simulink model "ModeleVehicule"  (R2018a)
settings: Solver=VariableStepAuto  StartTime=0.0  StopTime=1180  RelTol=1e-3
undefined symbols (not defined in the file or in its folder): cb, crr, cx, g, m, mlimit, nc, nm, nr, r, rho, rr, s
libraries: drivecyclelib x1
settings Model: Creator=Thomas  LastModifiedBy=Thomas

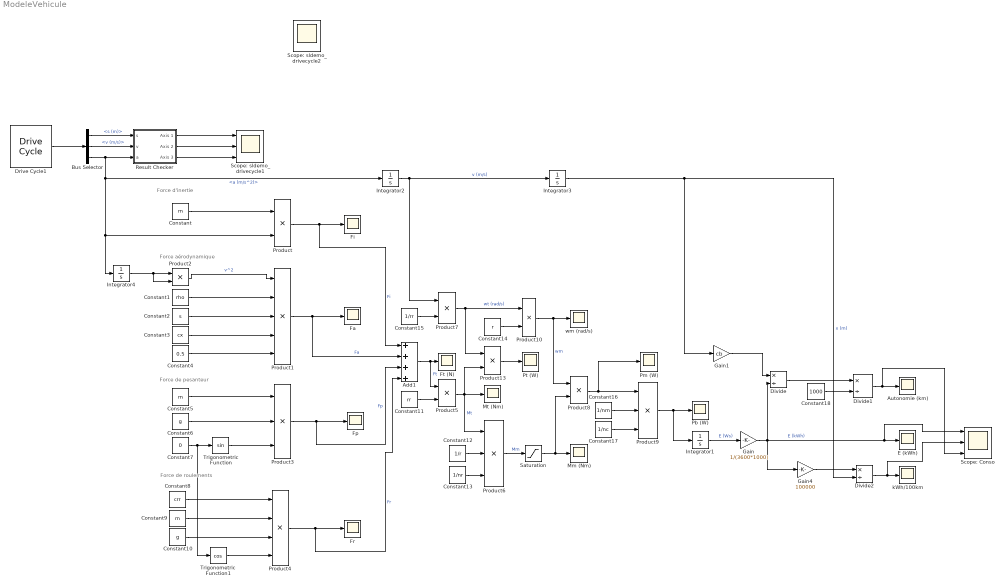
== system ModeleVehicule ==
  note: Force de pesanteur
  note: Force aérodynamique
  note: Force d'inertie
  note: Force de roulements
  Add1 : Sum  Inputs=++++
  Autonomie (km) : Scope
  Bus Selector : BusSelector  OutputSignals=s (m),v (m/s),a (m/s^2)
  Constant : Constant  Value=m
  Constant1 : Constant  Value=rho
  Constant10 : Constant  Value=g
  Constant11 : Constant  Value=rr
  Constant12 : Constant  Value=1/r
  Constant13 : Constant  Value=1/nr
  Constant14 : Constant  Value=r
  Constant15 : Constant  Value=1/rr
  Constant16 : Constant  Value=1/nm
  Constant17 : Constant  Value=1/nc
  Constant18 : Constant  Value=1000
  Constant2 : Constant  Value=s
  Constant3 : Constant  Value=cx
  Constant4 : Constant  Value=0.5
  Constant5 : Constant  Value=m
  Constant6 : Constant  Value=g
  Constant7 : Constant  Value=0
  Constant8 : Constant  Value=crr
  Constant9 : Constant  Value=m
  Divide : Product  Inputs=*/
  Divide1 : Product  Inputs=*/
  Divide2 : Product  Inputs=*/
  Drive Cycle1 : drivecyclelib/Drive Cycle  CycleName=NEDC  CycleRepeatsForever=off
      settings: SourceProductName=Drive Cycles Blockset
  E (kWh) : Scope
  Fa : Scope
  Fi : Scope
  Fp : Scope
  Fr : Scope
  Ft (N) : Scope
  Gain : Gain  Gain=1/(3600*1000)
  Gain1 : Gain  Gain=cb
  Gain4 : Gain  Gain=100000
  Integrator{1..4} (4 alike) : Integrator
  Mm (Nm) : Scope
  Mt (Nm) : Scope
  Pb (W) : Scope
  Pm (W) : Scope
  Product{,2,5,7..8,10,13} (7 alike) : Product
  Product1 : Product  Inputs=5
  Product3 : Product  Inputs=3
  Product4 : Product  Inputs=4
  Product6 : Product  Inputs=3
  Product9 : Product  Inputs=3
  Pt (W) : Scope
  Result Checker : Subsystem
  Saturation : Saturate  UpperLimit=mlimit  LowerLimit=-mlimit
  Scope: Conso : Scope  NumInputPorts=3
  Scope: sldemo_drivecycle1 : Scope  NumInputPorts=3
  Scope: sldemo_drivecycle2 : Scope  NumInputPorts=3
  Trigonometric Function : Trigonometry
  Trigonometric Function1 : Trigonometry  Operator=cos
  "kWh/100km " : Scope
  wm (rad/s) : Scope
  wires:
  Constant/1 -> Product/1
  Product/1 -> Fi/1, Add1/1  "Fi"
  Product2/1 -> Product1/1  "v^2"
  Constant1/1 -> Product1/2
  Constant2/1 -> Product1/3
  Constant3/1 -> Product1/4
  Product1/1 -> Add1/2, Fa/1  "Fa"
  Constant4/1 -> Product1/5
  Constant5/1 -> Product3/1
  Constant6/1 -> Product3/2
  Product3/1 -> Add1/3, Fp/1  "Fp"
  Constant8/1 -> Product4/1
  Constant10/1 -> Product4/3
  Constant9/1 -> Product4/2
  Product4/1 -> Add1/4, Fr/1  "Fr"
  Constant11/1 -> Product5/2
  Product5/1 -> Mt (Nm)/1, Product6/1, Product13/2  "Mt"
  Constant12/1 -> Product6/2
  Product7/1 -> Product10/1, Product13/1  "wt (rad/s)"
  Constant16/1 -> Product9/2
  Product9/1 -> Pb (W)/1, Integrator1/1
  Constant15/1 -> Product7/2
  Product10/1 -> Product8/1, wm (rad/s)/1  "wm"
  Constant14/1 -> Product10/2
  Integrator1/1 -> Gain/1  "E (Ws)"
  Gain/1 -> Divide/2, Scope: Conso/1, E (kWh)/1, Gain4/1  "E (kWh)"
  Divide/1 -> Divide1/1
  Gain1/1 -> Divide/1
  Bus Selector/1 -> Result Checker/1(s)  "<s (m)>"
  Drive Cycle1/1 -> Bus Selector/1
  Result Checker/2(Axis 2) -> Scope: sldemo_drivecycle1/2
  Bus Selector/3 -> Integrator2/1, Integrator4/1, Product/2, Result Checker/3(a)  "<a (m/s^2)>"
  Bus Selector/2 -> Result Checker/2(v)  "<v (m/s)>"
  Result Checker/1(Axis 1) -> Scope: sldemo_drivecycle1/1
  Result Checker/3(Axis 3) -> Scope: sldemo_drivecycle1/3
  Divide2/1 -> Scope: Conso/2, "kWh/100km "/1
  Trigonometric Function/1 -> Product3/3
  Trigonometric Function1/1 -> Product4/4
  Add1/1 -> Product5/1, Ft (N)/1  "Ft"
  Constant17/1 -> Product9/3
  Gain4/1 -> Divide2/1
  Integrator4/1 -> Product2/2, Product2/1
  Integrator2/1 -> Integrator3/1, Product7/1  "v (m/s)"
  Integrator3/1 -> Gain1/1, Divide2/2  "x (m)"
  Divide1/1 -> Autonomie (km)/1, Scope: Conso/3
  Constant18/1 -> Divide1/2
  Constant7/1 -> Trigonometric Function1/1, Trigonometric Function/1
  Constant13/1 -> Product6/3
  Product8/1 -> Pm (W)/1, Product9/1
  Product13/1 -> Pt (W)/1
  Product6/1 -> Saturation/1  "Mm"
  Saturation/1 -> Mm (Nm)/1, Product8/2

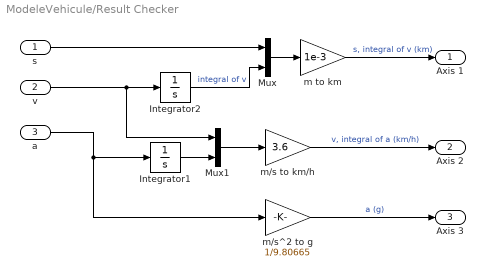
== system ModeleVehicule/Result Checker ==
  s : Inport
  v : Inport  Port=2
  a : Inport  Port=3
  Integrator1 : Integrator
  Integrator2 : Integrator
  Mux : Mux  Inputs=2
  Mux1 : Mux  Inputs=2
  m to km : Gain  Gain=1e-3
  m/s to km/h : Gain  Gain=3.6
  m/s^2 to g : Gain  Gain=1/9.80665
  Axis 1 : Outport
  Axis 2 : Outport  Port=2
  Axis 3 : Outport  Port=3
  wires:
  Mux/1 -> m to km/1
  Integrator1/1 -> Mux1/2
  Integrator2/1 -> Mux/2  "integral of v"
  Mux1/1 -> m/s to km/h/1
  v/1 -> Integrator2/1, Mux1/1
  a/1 -> m/s^2 to g/1, Integrator1/1
  s/1 -> Mux/1
  m to km/1 -> Axis 1/1  "s, integral of v (km)"
  m/s to km/h/1 -> Axis 2/1  "v, integral of a (km/h)"
  m/s^2 to g/1 -> Axis 3/1  "a (g)"
